simulink model "fcm"  (R2017b)
settings: Solver=FixedStepAuto  StartTime=0.0  StopTime=sim_time  FixedStep=time_step/10  RelTol=1e-3
values from neighbouring files (symbols this model uses):
  fcm = struct(fcm)    [constants17.m]    (also in constants18.m)
  setV = 0    [init.m]
  your_dut = 18    [init.m]
  Zs0 = [0 0 0 0]    [constants17.m]    (also in constants18.m)
undefined symbols (not defined in the file or in its folder): sigbuilder_block
libraries: simulink x2
settings Model: SimulationMode=accelerator  Creator=rvorster  LastModifiedBy=rvorster

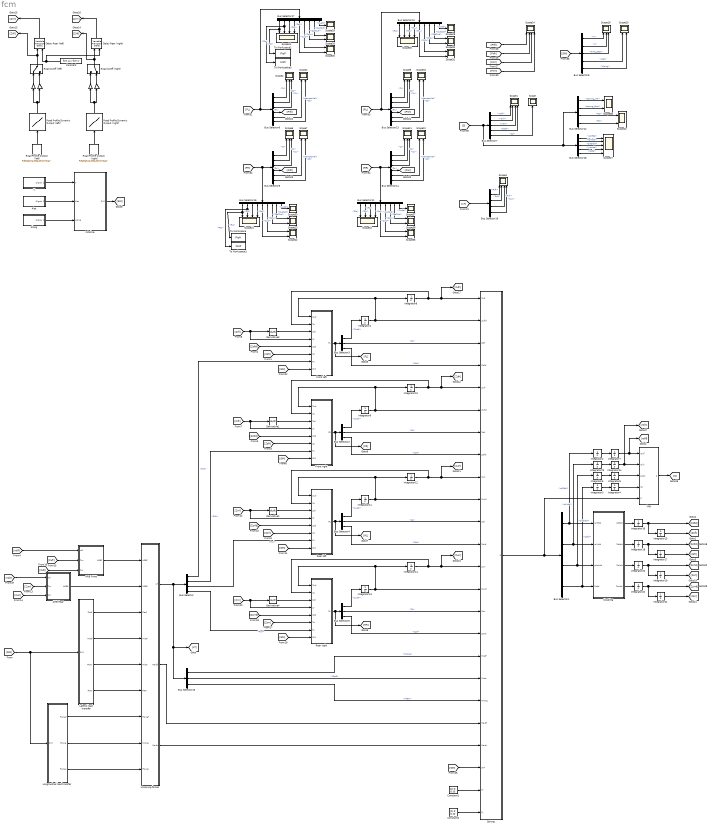
== system fcm ==
  " " : Gain
  " " : Gain  Gain=0
  " " : Gain  Gain=0
  " " : Gain
  "ARB Front " : MATLAB Function  TreatAsAtomicUnit=on
  ARB Rear : MATLAB Function  TreatAsAtomicUnit=on
  Alat : Subsystem  Tag=STV Subsys  LoadFcn=sigbuilder_block('load');  StartFcn=sigbuilder_block('start');  StopFcn=sigbuilder_block('stop');  ClipboardFcn=sigbuilder_block('clipboard');  mask(Sigbuilder block){tuvar=[0:10]}
      mask help: Simulink:masks:SigbuilderBlock_MD
      mask init:
      | if ~strcmp(get_param(bdroot(gcbh),'SimulationStatus'),'stopped') tuvar = sigbuilder_block('maskInit'); end
      settings: CopyFcn=sigbuilder_block('copy');  DeleteFcn=sigbuilder_block('delete');  ModelCloseFcn=sigbuilder_block('modelClose');  PreSaveFcn=sigbuilder_block('preSave');  PauseFcn=sigbuilder_block('pause');  ContinueFcn=sigbuilder_block('continue');  NameChangeFcn=sigbuilder_block('namechange');  OpenFcn=sigbuilder_block('open',[429.75 192 565.5 402.75 ]);  CloseFcn=sigbuilder_block('close');
      mask Display: plot(0, 0, 100, 100,[2, 2, 32, 32, 2], [68, 8, 8, 68, 68],[32, 2], [38, 38], [32, 19, 2],[53, 60, 44], [32, 17, 17, 2],[16, 16, 31, 31]);txt = getActiveGroup(gcbh);text(2, 100, txt,'verticalAlignment', 'top');
  Along : Subsystem  Tag=STV Subsys  LoadFcn=sigbuilder_block('load');  StartFcn=sigbuilder_block('start');  StopFcn=sigbuilder_block('stop');  ClipboardFcn=sigbuilder_block('clipboard');  mask(Sigbuilder block){tuvar=[0:10]}
      mask help: Simulink:masks:SigbuilderBlock_MD
      mask init:
      | if ~strcmp(get_param(bdroot(gcbh),'SimulationStatus'),'stopped') tuvar = sigbuilder_block('maskInit'); end
      settings: CopyFcn=sigbuilder_block('copy');  DeleteFcn=sigbuilder_block('delete');  ModelCloseFcn=sigbuilder_block('modelClose');  PreSaveFcn=sigbuilder_block('preSave');  PauseFcn=sigbuilder_block('pause');  ContinueFcn=sigbuilder_block('continue');  NameChangeFcn=sigbuilder_block('namechange');  OpenFcn=sigbuilder_block('open',[433.5 195.75 558 401.25 ]);  CloseFcn=sigbuilder_block('close');
      mask Display: plot(0, 0, 100, 100,[2, 2, 32, 32, 2], [68, 8, 8, 68, 68],[32, 2], [38, 38], [32, 19, 2],[53, 60, 44], [32, 17, 17, 2],[16, 16, 31, 31]);txt = getActiveGroup(gcbh);text(2, 100, txt,'verticalAlignment', 'top');
  Bus Selector : BusSelector  OutputSignals=Fufl,Fufr,Furl,Furr
  Bus Selector1 : BusSelector  OutputSignals=rollfdd,rollrdd,pitchdd,Zsdd
  Bus Selector{10..11,16..17} (4 alike) : BusSelector  OutputSignals=Fks,Fcs,Fku,Fcu,ZuZr,ZsZu,ZsdZud,ZudZrd,Zudd
  Bus Selector12 : BusSelector  OutputSignals=sprung_vel,sprung_disp,Fcs,Fks
  Bus Selector{6,9,13..14} (4 alike) : BusSelector  OutputSignals=Zr,Zs,Zu,Fn,damperVel,Cs
  Bus Selector15 : BusSelector  OutputSignals=Mlong,Mlatf,Mlatr
  Bus Selector18 : BusSelector  OutputSignals=rollfdd,rollrdd,pitchdd,yawdd,Zsdd
  Bus Selector19 : BusSelector  OutputSignals=Fufl,Fufr,Furl,Furr
  Bus Selector{2..5} (4 alike) : BusSelector  OutputSignals=Zudd,Zs,Zsd
  Bus Selector7 : BusSelector  OutputSignals=rollf,rollr,yaw,pitch,Zs
  Bus Selector8 : BusSelector  OutputSignals=V,L,time_step,Alat,Along
  Constant : Constant  Value=fcm.Lc / fcm.V
  Constant1 : Constant  Value=[0; 0; 0; 0]
  Constant2 : Constant  Value=[0; 0; 0; 0]
  Coupling : MATLAB Function  TreatAsAtomicUnit=on
  Delay Rear (left) : VariableTransportDelay  VariableDelayType=Variable transport delay  MaximumDelay=10  MaximumPoints=4096
  Delay Rear (right) : VariableTransportDelay  VariableDelayType=Variable transport delay  MaximumDelay=10  MaximumPoints=4096
  Derivative{1..4} (4 alike) : Derivative
  Front left : MATLAB Function  TreatAsAtomicUnit=on
  Front right : MATLAB Function  TreatAsAtomicUnit=on
  Initalize : MATLAB Function  TreatAsAtomicUnit=on
  Integrator{1..7,9,11,13,16,18,20,22..24} (16 alike) : Integrator
  Integrator10 : Integrator  InitialCondition=-Zs0(1)
  Integrator12 : Integrator  InitialCondition=-Zs0(3)
  Integrator14 : Integrator  InitialCondition=-Zs0(4)
  Integrator15 : Integrator  InitialCondition=-Zs0(1)
  Integrator17 : Integrator  InitialCondition=-Zs0(2)
  Integrator19 : Integrator  InitialCondition=-Zs0(3)
  Integrator21 : Integrator  InitialCondition=-Zs0(4)
  Integrator8 : Integrator  InitialCondition=-Zs0(1)
  Lateral load transfer : MATLAB Function  TreatAsAtomicUnit=on
  Log : MATLAB Function  TreatAsAtomicUnit=on
  "Longitudinal load transfer " : MATLAB Function  TreatAsAtomicUnit=on
  Rear left : MATLAB Function  TreatAsAtomicUnit=on
  Rear right : MATLAB Function  TreatAsAtomicUnit=on
  Road Profile Dynamic Output (left) : Lookup_n-D  NumberOfTableDimensions=1  BreakpointsForDimension1=[-5:5]  Table=tanh([-5:5])  InternalRulePriority=Speed  RndMeth=Simplest  InputSameDT=on
  Road Profile Dynamic Output (right) : Lookup_n-D  NumberOfTableDimensions=1  BreakpointsForDimension1=[-5:5]  Table=tanh([-5:5])  InternalRulePriority=Speed  RndMeth=Simplest  InputSameDT=on
  Road Profile Output (left) : simulink/Sources/Repeating Sequence Stair  OutValues=hx_left  tsamp=time_step  OutMin=[]  OutMax=[]  OutDataTypeStr=double  OutputDataTypeScalingMode=double  OutDataType=fixdt(0,8)  ConRadixGroup=Best Precision: Vector-wise  OutScaling=2^-12
  Road Profile Output (right) : simulink/Sources/Repeating Sequence Stair  OutValues=hx_right  tsamp=time_step  OutMin=[]  OutMax=[]  OutDataTypeStr=double  OutputDataTypeScalingMode=double  OutDataType=fixdt(0,8)  ConRadixGroup=Best Precision: Vector-wise  OutScaling=2^-12
  Road on/off (left) : ManualSwitch
  Road on/off (right) : ManualSwitch  CurrentSetting=0
  Scope{,28..29,33,37} (5 alike) : Scope
  Scope{1,3,14,21,24,30,34} (7 alike) : Scope  NumInputPorts=4
  Scope{2,6,9,11,19} (5 alike) : Scope  NumInputPorts=3
  Scope{4,7,12,18,20,22..23,25..26,31..32,35..36,38,40} (15 alike) : Scope  NumInputPorts=2
  Scope27 : Scope  NumInputPorts=5
  Sprung : MATLAB Function  TreatAsAtomicUnit=on
  To Workspace : ToWorkspace  VariableName=Fksfr  SaveFormat=Timeseries  SampleTime=-1
  To Workspace1 : ToWorkspace  VariableName=Fcsfr  SaveFormat=Timeseries  SampleTime=-1
  To Workspace2 : ToWorkspace  VariableName=Fksfl  SaveFormat=Timeseries  SampleTime=-1
  To Workspace3 : ToWorkspace  VariableName=Fcsfl  SaveFormat=Timeseries  SampleTime=-1
  Unsprung forces : MATLAB Function  TreatAsAtomicUnit=on
  V : Subsystem  Tag=STV Subsys  LoadFcn=sigbuilder_block('load');  StartFcn=sigbuilder_block('start');  StopFcn=sigbuilder_block('stop');  ClipboardFcn=sigbuilder_block('clipboard');  mask(Sigbuilder block){tuvar=[0:10]}
      mask help: Simulink:masks:SigbuilderBlock_MD
      mask init:
      | if ~strcmp(get_param(bdroot(gcbh),'SimulationStatus'),'stopped') tuvar = sigbuilder_block('maskInit'); end
      settings: CopyFcn=sigbuilder_block('copy');  DeleteFcn=sigbuilder_block('delete');  ModelCloseFcn=sigbuilder_block('modelClose');  PreSaveFcn=sigbuilder_block('preSave');  PauseFcn=sigbuilder_block('pause');  ContinueFcn=sigbuilder_block('continue');  NameChangeFcn=sigbuilder_block('namechange');  OpenFcn=sigbuilder_block('open',[433.5 195.75 558 401.25 ]);  CloseFcn=sigbuilder_block('close');
      mask Display: plot(0, 0, 100, 100,[2, 2, 32, 32, 2], [68, 8, 8, 68, 68],[32, 2], [38, 38], [32, 19, 2],[53, 60, 44], [32, 17, 17, 2],[16, 16, 31, 31]);txt = getActiveGroup(gcbh);text(2, 100, txt,'verticalAlignment', 'top');
  wires:
  Lateral load transfer/1(Flatf) -> Unsprung forces/3(Flatf)
  Integrator6/1 -> Log/3(pitch)
  Constant2/1 -> Sprung/24(Fy)
  Constant1/1 -> Sprung/23(Fx)
  Integrator7/1 -> Log/1(rollf), [rollf]
  "Longitudinal load transfer "/3(Flongr) -> Unsprung forces/9(Flongr)
  [rollf] -> "ARB Front "/1(roll)
  Integrator4/1 -> Log/4(Zs)
  "Longitudinal load transfer "/1(Flongf) -> Unsprung forces/7(Flongf)
  Lateral load transfer/2(Mlatf) -> Unsprung forces/4(Mlatf)
  Lateral load transfer/4(Flatr) -> Unsprung forces/6(Flatr)
  Coupling/1(Zsfldd) -> Integrator16/1
  "Longitudinal load transfer "/2(Mlong) -> Unsprung forces/8(Mlong)
  Delay Rear (right)/1 -> [Zrrr]
  Along/1(Signal 1) -> Initalize/3(Along)
  V/1(Signal 1) -> Initalize/1(V)
  Road Profile Output (left)/1 -> Road Profile Dynamic Output (left)/1
  " "/1 -> Road on/off (right)/2
  " "/1 -> Road on/off (right)/1
  Road on/off (right)/1 -> [Zrfr], Delay Rear (right)/1
  Road on/off (left)/1 -> [Zrfl], Delay Rear (left)/1
  Alat/1(Signal 1) -> Initalize/2(Alat)
  Constant/1 -> Delay Rear (right)/2, Delay Rear (left)/2
  " "/1 -> Road on/off (left)/2
  Road Profile Output (right)/1 -> Road Profile Dynamic Output (right)/1
  Road Profile Dynamic Output (left)/1 -> " "/1, " "/1
  " "/1 -> Road on/off (left)/1
  Road Profile Dynamic Output (right)/1 -> " "/1, " "/1
  Sprung/1(S) -> Log/5("S "), Bus Selector1/1
  Integrator2/1 -> Integrator7/1
  Integrator5/1 -> Integrator6/1
  Integrator3/1 -> Integrator4/1
  "ARB Front "/1(ARBF) -> Unsprung forces/1(ARBF)
  ARB Rear/1(ARBR) -> Unsprung forces/2(ARBR)
  [Zufl] -> "ARB Front "/3(Zul)
  [Zurr] -> ARB Rear/2(Zur)
  [Zurl] -> ARB Rear/3(Zul)
  [Zufr] -> "ARB Front "/2(Zur)
  Unsprung forces/2(Marbf) -> Sprung/20(Marbf)
  Unsprung forces/3(Marbr) -> Sprung/21(Marbr)
  Initalize/1(SIM) -> [SIM]
  [SIM] -> "Longitudinal load transfer "/1(SIM), Lateral load transfer/1(SIM)
  [SIM] -> Sprung/22(SIM)
  Bus Selector10/2 -> Scope30/2  "<Fcs>"
  [Fnrr] -> Scope14/4
  Bus Selector14/3 -> Scope11/3  "<Zu>"
  Bus Selector16/5 -> Scope22/2  "<ZuZr>"
  Bus Selector10/3 -> Scope30/3  "<Fku>"
  Bus Selector7/1 -> Scope1/1  "<rollf>"
  Bus Selector8/4 -> Scope20/1  "<Alat>"
  Bus Selector9/5 -> Scope7/1  "<damperVel>"
  Bus Selector11/4 -> Scope34/4  "<Fcu>"
  Bus Selector17/1 -> To Workspace2/1, Scope24/1  "<Fks>"
  Bus Selector10/8 -> Scope32/1  "<ZudZrd>"
  Bus Selector13/1 -> Scope9/1  "<Zr>"
  Bus Selector17/3 -> Scope24/3  "<Fku>"
  Bus Selector17/8 -> Scope26/1  "<ZudZrd>"
  Bus Selector12/3 -> Scope40/1  "<Fcs>"
  Bus Selector17/5 -> Scope25/2  "<ZuZr>"
  Bus Selector17/7 -> Scope26/2  "<ZsdZud>"
  [FL] -> Bus Selector17/1, Bus Selector6/1
  Bus Selector17/2 -> To Workspace3/1, Scope24/2  "<Fcs>"
  Bus Selector10/7 -> Scope32/2  "<ZsdZud>"
  Bus Selector6/1 -> Scope2/1  "<Zr>"
  Bus Selector16/8 -> Scope23/1  "<ZudZrd>"
  Bus Selector16/7 -> Scope23/2  "<ZsdZud>"
  Bus Selector13/3 -> Scope9/3  "<Zu>"
  [Fnrl] -> Scope14/3
  Bus Selector16/6 -> Scope22/1  "<ZsZu>"
  Bus Selector8/1 -> Scope19/1  "<V>"
  Bus Selector16/4 -> Scope21/4  "<Fcu>"
  Bus Selector14/1 -> Scope11/1  "<Zr>"
  Bus Selector16/2 -> To Workspace1/1, Scope21/2  "<Fcs>"
  Bus Selector13/5 -> Scope18/1  "<damperVel>"
  Bus Selector16/3 -> Scope21/3  "<Fku>"
  Bus Selector11/9 -> Scope37/1  "<Zudd>"
  [Fnfl] -> Scope14/1
  Bus Selector8/3 -> Scope19/3  "<time_step>"
  Bus Selector10/6 -> Scope31/1  "<ZsZu>"
  [SIM] -> Bus Selector8/1
  Bus Selector9/4 -> [Fnfr]  "<Fn>"
  Bus Selector11/8 -> Scope36/1  "<ZudZrd>"
  Bus Selector11/3 -> Scope34/3  "<Fku>"
  Bus Selector9/6 -> Scope7/2  "<Cs>"
  Bus Selector9/2 -> Scope6/2  "<Zs>"
  Bus Selector6/5 -> Scope4/1  "<damperVel>"
  Bus Selector6/3 -> Scope2/3  "<Zu>"
  Bus Selector9/1 -> Scope6/1  "<Zr>"
  Bus Selector18/5 -> Scope27/5  "<Zsdd>"
  Bus Selector7/3 -> Scope1/3  "<yaw>"
  Bus Selector7/4 -> Scope1/4  "<pitch>"
  Bus Selector14/5 -> Scope12/1  "<damperVel>"
  Bus Selector18/1 -> Scope27/1  "<rollfdd>"
  [RL] -> Bus Selector10/1, Bus Selector13/1
  Bus Selector6/4 -> [Fnfl]  "<Fn>"
  Bus Selector14/2 -> Scope11/2  "<Zs>"
  Bus Selector13/2 -> Scope9/2  "<Zs>"
  Bus Selector18/4 -> Scope27/4  "<yawdd>"
  Bus Selector14/6 -> Scope12/2  "<Cs>"
  Bus Selector6/6 -> Scope4/2  "<Cs>"
  Bus Selector14/4 -> [Fnrr]  "<Fn>"
  Bus Selector12/4 -> Scope40/2  "<Fks>"
  Bus Selector13/4 -> [Fnrl]  "<Fn>"
  Bus Selector18/3 -> Scope27/3  "<pitchdd>"
  [Fnfr] -> Scope14/2
  Bus Selector10/4 -> Scope30/4  "<Fcu>"
  Bus Selector13/6 -> Scope18/2  "<Cs>"
  Bus Selector17/9 -> Scope29/1  "<Zudd>"
  Bus Selector16/1 -> To Workspace/1, Scope21/1  "<Fks>"
  Bus Selector17/4 -> Scope24/4  "<Fcu>"
  Bus Selector9/3 -> Scope6/3  "<Zu>"
  Bus Selector11/7 -> Scope36/2  "<ZsdZud>"
  [RR] -> Bus Selector14/1, Bus Selector11/1
  Bus Selector10/1 -> Scope30/1  "<Fks>"
  [FR] -> Bus Selector9/1, Bus Selector16/1
  Bus Selector11/2 -> Scope34/2  "<Fcs>"
  Bus Selector8/2 -> Scope19/2  "<L>"
  Bus Selector10/9 -> Scope28/1  "<Zudd>"
  Bus Selector11/6 -> Scope35/1  "<ZsZu>"
  Bus Selector11/5 -> Scope35/2  "<ZuZr>"
  Bus Selector12/1 -> Scope38/1  "<sprung_vel>"
  Bus Selector12/2 -> Scope38/2  "<sprung_disp>"
  Bus Selector10/5 -> Scope31/2  "<ZuZr>"
  Bus Selector11/1 -> Scope34/1  "<Fks>"
  Bus Selector17/6 -> Scope25/1  "<ZsZu>"
  Bus Selector16/9 -> Scope33/1  "<Zudd>"
  Bus Selector8/5 -> Scope20/2  "<Along>"
  Bus Selector6/2 -> Scope2/2  "<Zs>"
  [S] -> Bus Selector7/1, Bus Selector12/1, Bus Selector18/1
  Log/1(S) -> [S]
  Bus Selector7/5 -> Scope/1  "<Zs>"
  Integrator23/1 -> Integrator24/1
  Bus Selector1/1 -> Integrator2/1, Coupling/1(rollfdd)  "<rollfdd>"
  Bus Selector1/2 -> Integrator23/1, Coupling/2(rollrdd)  "<rollrdd>"
  Bus Selector1/3 -> Integrator5/1, Coupling/3(pitchdd)  "<pitchdd>"
  Bus Selector1/4 -> Integrator3/1, Coupling/4(Zsdd)  "<Zsdd>"
  Lateral load transfer/3(Mlatr) -> Unsprung forces/5(Mlatr)
  Bus Selector7/2 -> Scope1/2  "<rollr>"
  Integrator24/1 -> [rollr], Log/2(rollr)
  [rollr] -> ARB Rear/1(roll)
  Bus Selector18/2 -> Scope27/2  "<rollrdd>"
  Bus Selector3/3 -> Sprung/4(Zsfld)  "<Zsd>"
  Bus Selector3/1 -> Integrator1/1  "<Zudd>"
  Bus Selector3/2 -> Sprung/3(Zsfl)  "<Zs>"
  Front left/1(FL) -> [FL], Bus Selector3/1
  [Zsfld] -> Front left/5(Zsd)
  [SIM] -> Front left/8(SIM)
  [Zrfl] -> Front left/4(Zr), Derivative3/1
  [Zsfl] -> Front left/6(Zs)
  Derivative3/1 -> Front left/3(Zrd)
  Integrator1/1 -> Sprung/2(Zufld), Integrator8/1, Front left/1(Zud)
  [Zsfr] -> Front right/6(Zs)
  Derivative1/1 -> Front right/3(Zrd)
  [Zsfrd] -> Front right/5(Zsd)
  Integrator9/1 -> Sprung/6(Zufrd), Integrator10/1, Front right/1(Zud)
  Bus Selector2/2 -> Sprung/7(Zsfr)  "<Zs>"
  Front right/1(FR) -> [FR], Bus Selector2/1
  [SIM] -> Front right/8(SIM)
  Bus Selector2/3 -> Sprung/8(Zsfrd)  "<Zsd>"
  Bus Selector2/1 -> Integrator9/1  "<Zudd>"
  [Zrfr] -> Front right/4(Zr), Derivative1/1
  [Zsrl] -> Rear left/6(Zs)
  Derivative2/1 -> Rear left/3(Zrd)
  [Zsrld] -> Rear left/5(Zsd)
  Integrator11/1 -> Sprung/10(Zurld), Integrator12/1, Rear left/1(Zud)
  Bus Selector4/2 -> Sprung/11(Zsrl)  "<Zs>"
  Rear left/1(RL) -> [RL], Bus Selector4/1
  [SIM] -> Rear left/8(SIM)
  Bus Selector4/3 -> Sprung/12(Zsrld)  "<Zsd>"
  Bus Selector4/1 -> Integrator11/1  "<Zudd>"
  [Zrrl] -> Rear left/4(Zr), Derivative2/1
  Integrator14/1 -> [Zurr], Sprung/13(Zurr), Rear right/2(Zu)
  [Zsrr] -> Rear right/6(Zs)
  Derivative4/1 -> Rear right/3(Zrd)
  [Zsrrd] -> Rear right/5(Zsd)
  Integrator13/1 -> Sprung/14(Zurrd), Integrator14/1, Rear right/1(Zud)
  Bus Selector5/2 -> Sprung/15(Zsrr)  "<Zs>"
  Rear right/1(FL) -> [RR], Bus Selector5/1
  [SIM] -> Rear right/8(SIM)
  Bus Selector5/3 -> Sprung/16(Zsrrd)  "<Zsd>"
  Bus Selector5/1 -> Integrator13/1  "<Zudd>"
  [Zrrr] -> Rear right/4(Zr), Derivative4/1
  Integrator12/1 -> [Zurl], Sprung/9(Zurl), Rear left/2(Zu)
  Integrator10/1 -> [Zufr], Sprung/5(Zufr), Front right/2(Zu)
  Integrator8/1 -> Front left/2(Zu), [Zufl], Sprung/1(Zufl)
  Integrator15/1 -> [Zsfl]
  Integrator16/1 -> [Zsfld], Integrator15/1
  Integrator17/1 -> [Zsfr]
  Integrator18/1 -> [Zsfrd], Integrator17/1
  Coupling/2(Zsfrdd) -> Integrator18/1
  Integrator19/1 -> [Zsrl]
  Integrator20/1 -> [Zsrld], Integrator19/1
  Coupling/3(Zsrldd) -> Integrator20/1
  Integrator21/1 -> [Zsrr]
  Integrator22/1 -> [Zsrrd], Integrator21/1
  Coupling/4(Zsrrdd) -> Integrator22/1
  Unsprung forces/1(LT) -> [LT], Bus Selector15/1, Bus Selector/1
  Bus Selector/4 -> Rear right/7(Fu)  "<Furr>"
  Bus Selector/3 -> Rear left/7(Fu)  "<Furl>"
  Bus Selector/2 -> Front right/7(Fu)  "<Fufr>"
  Bus Selector/1 -> Front left/7(Fu)  "<Fufl>"
  Bus Selector15/2 -> Sprung/18(Mlatr)  "<Mlatf>"
  Bus Selector15/1 -> Sprung/17(Mlatf)  "<Mlong>"
  Bus Selector15/3 -> Sprung/19(Mlong)  "<Mlatr>"
  [LT] -> Bus Selector19/1
  Bus Selector19/1 -> Scope3/1  "<Fufl>"
  Bus Selector19/2 -> Scope3/2  "<Fufr>"
  Bus Selector19/3 -> Scope3/3  "<Furl>"
  Bus Selector19/4 -> Scope3/4  "<Furr>"
  Delay Rear (left)/1 -> [Zrrl]

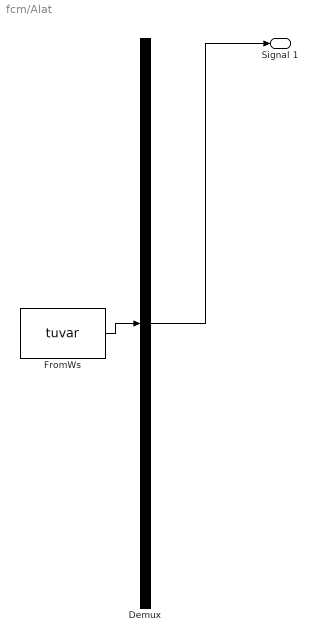
== system fcm/Alat ==
  Demux : Demux  Tag=STV Demux  Outputs=1
  FromWs : FromWorkspace  Tag=STV FromWs  VariableName=tuvar  SampleTime=0
      SigBuilderData=|
      | common.afterFinalStr = 'Extrapolate'
      | common.sampleTime = 0
      | dataSet.timeRange = [0 10]
      | dataSet.name = 'Group 1'
      | sbobj.Groups.Name = 'Group 1'
      | sbobj.Groups.Signals.Name = 'Signal 1'
      | sbobj.Groups.Signals.XData = [0 4 6 10]
      | sbobj.Groups.Signals.YData = [0 0 0 0]
  Signal 1 : Outport  Tag=STV Outport
  wires:
  Demux/1 -> Signal 1/1
  FromWs/1 -> Demux/1

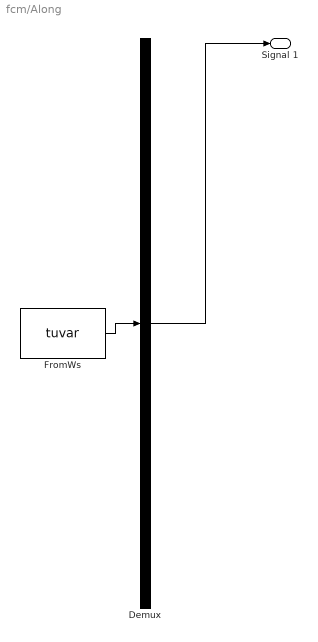
== system fcm/Along ==
  Demux : Demux  Tag=STV Demux  Outputs=1
  FromWs : FromWorkspace  Tag=STV FromWs  VariableName=tuvar  SampleTime=0
      SigBuilderData=|
      | common.afterFinalStr = 'Extrapolate'
      | common.sampleTime = 0
      | dataSet.timeRange = [0 10]
      | dataSet.name = 'Group 1'
      | sbobj.Groups.Name = 'Group 1'
      | sbobj.Groups.Signals.Name = 'Signal 1'
      | sbobj.Groups.Signals.XData = [0 4 4 6 6 10]
      | sbobj.Groups.Signals.YData = [0 0 0 0 0 0]
  Signal 1 : Outport  Tag=STV Outport
  wires:
  Demux/1 -> Signal 1/1
  FromWs/1 -> Demux/1

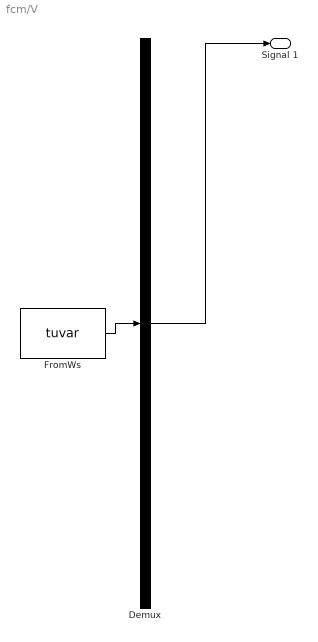
== system fcm/V ==
  Demux : Demux  Tag=STV Demux  Outputs=1
  FromWs : FromWorkspace  Tag=STV FromWs  VariableName=tuvar  SampleTime=0
      SigBuilderData=|
      | common.afterFinalStr = 'Extrapolate'
      | common.sampleTime = 0
      | dataSet.timeRange = [0 10]
      | dataSet.name = 'Group 1'
      | sbobj.Groups.Name = 'Group 1'
      | sbobj.Groups.Signals.Name = 'Signal 1'
      | sbobj.Groups.Signals.XData = [0 4 6 10]
      | sbobj.Groups.Signals.YData = [0 35 0 0]
  Signal 1 : Outport  Tag=STV Outport
  wires:
  Demux/1 -> Signal 1/1
  FromWs/1 -> Demux/1

== matlab function fcm/Front right ==
  data: Zud input; Zu input; Zrd input; Zr input; Zsd input; Zs input; Fu input; fcm parameter; FR output Bus: U; SIM input Bus: SIM; Zs0 parameter
function FR = fcn(Zud, Zu, Zrd, Zr, Zsd, Zs, Fu, fcm, SIM, Zs0)

    loc = 2;
    FR = unsprung_mass(Zud, Zu, Zrd, Zr, Zsd, Zs, Fu, loc, SIM, Zs0, fcm);

end

== matlab function fcm/Rear left ==
  data: Zud input; Zu input; Zrd input; Zr input; Zsd input; Zs input; Fu input; fcm parameter; RL output Bus: U; SIM input Bus: SIM; Zs0 parameter
function RL = fcn(Zud, Zu, Zrd, Zr, Zsd, Zs, Fu, fcm, SIM, Zs0)

    loc = 3;
    RL = unsprung_mass(Zud, Zu, Zrd, Zr, Zsd, Zs, Fu, loc, SIM, Zs0, fcm);

end

== matlab function fcm/Log ==
  data: rollf input; rollr input; S output; pitch input; Zs input; S input Bus: C
function S = fcn(rollf, rollr, pitch, Zs, S)

    S.rollf = rollf;
    S.rollr = rollr;
    S.pitch = pitch;
    S.Zs = Zs;
    
end

== matlab function fcm/Front left ==
  data: Zud input; Zu input; Zrd input; Zr input; Zsd input; Zs input; Fu input; fcm parameter; FL output Bus: U; SIM input Bus: SIM; Zs0 parameter
function FL = fcn(Zud, Zu, Zrd, Zr, Zsd, Zs, Fu, fcm, SIM, Zs0)

    loc = 1;
    FL = unsprung_mass(Zud, Zu, Zrd, Zr, Zsd, Zs, Fu, loc, SIM, Zs0, fcm);

end

== matlab function fcm/Sprung ==
  data: Zufl input; Zufld input; Zsfl input; Zsfld input; Zufr input; Zufrd input; Zsfr input; Zsfrd input; Zurl input; Zurld input; Zsrl input; Zsrld input; Zurr input; Zurrd input; Zsrr input; Zsrrd input; Mlatf input; Mlatr input; Mlong input; Marbf input; Marbr input; SIM input Bus: SIM; Fx input; Fy input; S output Bus: C; fcm parameter
function S  = fcn(Zufl, Zufld, Zsfl, Zsfld, Zufr, Zufrd, Zsfr, Zsfrd, Zurl, Zurld, Zsrl, Zsrld, Zurr, Zurrd, Zsrr, Zsrrd, Mlatf, Mlatr, Mlong, Marbf, Marbr, SIM, Fx, Fy, fcm)

    S = sprung_mass(Zufl, Zufld, Zsfl, Zsfld, Zufr, Zufrd, Zsfr, Zsfrd, ...
        Zurl, Zurld, Zsrl, Zsrld, Zurr, Zurrd, Zsrr, Zsrrd, Mlatf, Mlatr, ...
        Mlong, Marbf, Marbr, SIM, Fx, Fy, fcm);

end

== matlab function fcm/Coupling ==
  data: rollfdd input; rollrdd input; Zsfldd output; Zsfrdd output; Zsrldd output; Zsrrdd output; pitchdd input; Zsdd input; fcm parameter
function [Zsfldd, Zsfrdd, Zsrldd, Zsrrdd] = fcn(rollfdd, rollrdd, pitchdd, Zsdd, fcm)

    [Zsfldd, Zsfrdd, Zsrldd, Zsrrdd] = coupling(rollfdd, rollrdd, pitchdd, Zsdd, fcm);
    
end

== matlab function fcm/ARB Front  ==
  settings: updateMethod=DISCRETE
  data: roll input; Zur input; Zul input; fcm parameter; ARBF output Bus: ARB
function ARBF = fcn(roll, Zur, Zul, fcm)

    loc = 0; % Front
    ARBF = arb(Zur, Zul, roll, loc, fcm);
    
end

== matlab function fcm/ARB Rear ==
  settings: updateMethod=DISCRETE
  data: roll input; ARBR output Bus: ARB; Zur input; Zul input; fcm parameter
function ARBR = fcn(roll, Zur, Zul, fcm)

    loc = 1; % Rear
    ARBR = arb(Zur, Zul, roll, loc, fcm);

end

== matlab function fcm/Lateral load transfer ==
  data: Flatf output; Mlatf output; Mlatr output; Flatr output; fcm parameter; SIM input Bus: SIM
function [Flatf, Mlatf, Mlatr, Flatr] = fcn(fcm, SIM)
    
    Alat = SIM.Alat;
    
    [Flatf, Mlatf, Mlatr, Flatr] = lateral_load(Alat, fcm);
    
end

== matlab function fcm/Longitudinal load transfer  ==
  data: Flongf output; Mlong output; Flongr output; fcm parameter; SIM input Bus: SIM
function [Flongf, Mlong, Flongr] = fcn(fcm, SIM)

    Along = SIM.Along;
    
    [Flongf, Mlong, Flongr] = longitudinal_load(Along, fcm);

end

== matlab function fcm/Unsprung forces ==
  data: ARBF input; ARBR input; Flatf input; Mlatf input; Mlatr input; Flatr input; Flongf input; Mlong input; Flongr input; LT output Bus: LT; Marbf output; Marbr output
function [LT, Marbf, Marbr] = fcn(ARBF, ARBR, Flatf, Mlatf, Mlatr, Flatr, Flongf, Mlong, Flongr)
    
    LT.Flatf = Flatf;
    LT.Flatr = Flatr;
    LT.Flongf = Flongf;
    LT.Flongr = Flongr;
    
    LT.Mlong = Mlong;
    LT.Mlatf = Mlatf;
    LT.Mlatr = Mlatr;
    
    LT.Fufl = Flongf - ARBF.Farb - Flatf;
    LT.Fufr = Flongf + ARBF.Farb + Flatf;
    LT.Furl = Flongr - ARBR.Farb - Flatr;
    LT.Furr = Flongr + ARBR.Farb + Flatr;
    
    Marbf = ARBF.Marb;
    Marbr = ARBR.Marb;
    
end

== matlab function fcm/Rear right ==
  data: Zud input; Zu input; Zrd input; Zr input; Zsd input; Zs input; Fu input; fcm parameter; FL output Bus: U; SIM input Bus: SIM; Zs0 parameter
function FL = fcn(Zud, Zu, Zrd, Zr, Zsd, Zs, Fu, fcm, SIM, Zs0)

    loc = 1;
    FL = unsprung_mass(Zud, Zu, Zrd, Zr, Zsd, Zs, Fu, loc, SIM, Zs0, fcm);

end

== matlab function fcm/Initalize ==
  settings: updateMethod=DISCRETE
  data: V input; Alat input; Along input; fcm parameter; SIM output Bus: SIM; setV parameter; your_dut parameter
function SIM = fcn(V, Alat, Along, fcm, setV, your_dut)

    if (setV == 0)
        SIM.V = fcm.V;
        SIM.L = 0.5*fcm.V^2*fcm.ClA*fcm.rho0;
        SIM.Alat = fcm.Alat;
        SIM.Along = fcm.Along;
        SIM.sim_time = 0;
        SIM.sim_step = 0;
        SIM.time_step = 0.01 / fcm.V;
        SIM.your_dut = your_dut;
    else
        SIM.V = V;
        SIM.L = 0.5*V^2*fcm.ClA*fcm.rho0;
        SIM.Alat = Alat;
        SIM.Along = Along;
        SIM.sim_time = 0;
        SIM.sim_step = 0;
        SIM.time_step = 0.01 / V;
        SIM.your_dut = your_dut;
    end

end
